simulink model "IMU2"  (R2018b)
settings: Solver=FixedStepAuto  StartTime=0.0  StopTime=inf  RelTol=1e-3  EnableMultiTasking=on
InitFcn:
  | Ts=0.1;
  | Delay=5;
  | Sample_div=uint8(9);
  | Filter_BW=uint8(2);  %cutoff 92 Hz
  | Gy_Conf=uint8(0); %-250dps to 250 dps
  | Acc_Conf1=uint8(0);
  | Acc_Conf2=uint8(2);
  | FIFO_en=uint8(0); % Disabled
  | INT_en=uint8(0); % Disabled
  | Acc_Scale=2*9.81/32767;
  | 
  | %Registers
  | IMU_Add=104;
  | Who_Am_I=117;
  | PWR_1=107;
  | PWR_2=108;
  | SAMPL_DIV=25;
  | CONFIG_REG=26;
  | GYRO_CONFIG=27;
  | ACC_CONFIG_1=28;
  | ACC_CONFIG_2=29;
  | FIFO_EN=35;
  | INT_EN=56;
  | GY_X_OFFSET_H=19;
  | GY_X_OFFSET_L=20;
  | GY_Y_OFFSET_H=21;
  | GY_Y_OFFSET_L=22;
  | GY_Z_OFFSET_H=23;
  | GY_Z_OFFSET_L=24;
  | ACC_X_OFFSET_H=119;
  | ACC_X_OFFSET_L=120;
  | ACC_Y_OFFSET_H=122;
  | ACC_Y_OFFSET_L=123;
  | ACC_Z_OFFSET_H=125;
  | ACC_Z_OFFSET_L=126;
  | ACCEL_XOUT_H=59;
  | ACCEL_XOUT_L=60;
  | ACCEL_YOUT_H=61;
  | ACCEL_YOUT_L=62;
  | ACCEL_ZOUT_H=63;
  | ACCEL_ZOUT_L=64
libraries: arduinolib x14
settings Model: SimulationMode=external  ExtModeTrigDuration=2  Creator=amind  LastModifiedBy=PC WORLD
settings OptimizationCC: EnhancedBackFolding=on  PassReuseOutputArgsAs=Individual arguments  MaxStackSize=64  OptimizeBlockOrder=speed  DifferentSizesBufferReuse=on  OptimizationCustomize=off
settings DebuggingCC: ParameterPrecisionLossMsg=none  ParameterTunabilityLossMsg=error
settings HardwareCC: ProdBitPerInt=16  ProdBitPerPointer=16  ProdBitPerSizeT=16  ProdBitPerPtrDiffT=16  ProdLargestAtomicFloat=None  ProdWordSize=8  ProdHWDeviceType=Atmel->AVR
settings SFSimCC: MATLABDynamicMemAlloc=off
settings RTWCC: SystemTargetFile=ert.tlc  HardwareBoard=Arduino Mega 2560  TemplateMakefile=ert_default_tmf  GenerateReport=on  Toolchain=Arduino AVR  BuildConfiguration=Faster Runs  IncludeHyperlinkInReport=on  LaunchReport=on  GenerateTraceInfo=on  GenerateTraceReport=on  GenerateTraceReportSl=on  GenerateTraceReportSf=on  GenerateTraceReportEml=on
settings CodeAppCC: ForceParamTrailComments=on  IgnoreCustomStorageClasses=off  OperatorAnnotations=on  SimulinkDataObjDesc=on  SFDataObjDesc=on  InsertBlockDesc=on
settings ERTTargetCC: SupportContinuousTime=on  SupportVariableSizeSignals=on

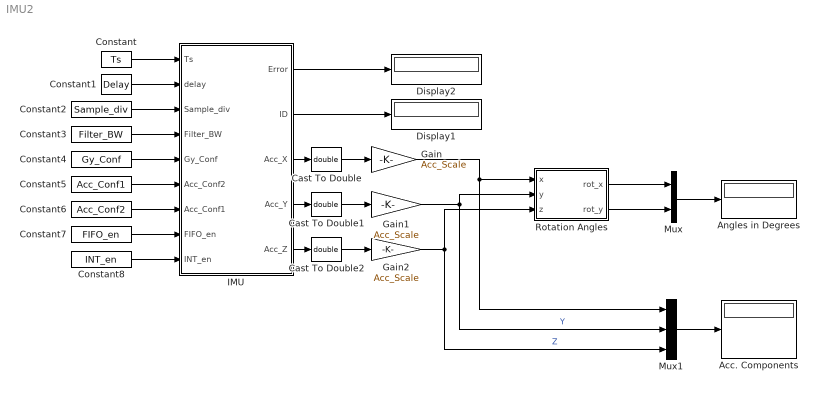
== system IMU2 ==
  Acc. Components : Display
  Angles in Degrees : Display
  Cast To Double : DataTypeConversion  OutDataTypeStr=double
  Cast To Double1 : DataTypeConversion  OutDataTypeStr=double
  Cast To Double2 : DataTypeConversion  OutDataTypeStr=double
  Constant : Constant  Value=Ts
  Constant1 : Constant  Value=Delay
  Constant2 : Constant  Value=Sample_div
  Constant3 : Constant  Value=Filter_BW
  Constant4 : Constant  Value=Gy_Conf
  Constant5 : Constant  Value=Acc_Conf1
  Constant6 : Constant  Value=Acc_Conf2
  Constant7 : Constant  Value=FIFO_en
  Constant8 : Constant  Value=INT_en
  Display1 : Display
  Display2 : Display
  Gain : Gain  Gain=Acc_Scale
  Gain1 : Gain  Gain=Acc_Scale
  Gain2 : Gain  Gain=Acc_Scale
  IMU : Stateflow chart  TreatAsAtomicUnit=on
  Mux : Mux  Inputs=2
  Mux1 : Mux  Inputs=3
  Rotation Angles : MATLAB Function  TreatAsAtomicUnit=on
  wires:
  IMU/1(Error) -> Display2/1
  IMU/2(ID) -> Display1/1
  Constant/1 -> IMU/1(Ts)
  Constant1/1 -> IMU/2(delay)
  Constant2/1 -> IMU/3(Sample_div)
  Constant3/1 -> IMU/4(Filter_BW)
  Constant4/1 -> IMU/5(Gy_Conf)
  Constant5/1 -> IMU/6(Acc_Conf2)
  Constant6/1 -> IMU/7(Acc_Conf1)
  Constant7/1 -> IMU/8(FIFO_en)
  Constant8/1 -> IMU/9(INT_en)
  IMU/3(Acc_X) -> Cast To Double/1
  IMU/4(Acc_Y) -> Cast To Double1/1
  IMU/5(Acc_Z) -> Cast To Double2/1
  Mux/1 -> Angles in Degrees/1
  Cast To Double/1 -> Gain/1
  Cast To Double1/1 -> Gain1/1
  Cast To Double2/1 -> Gain2/1
  Gain/1 -> Rotation Angles/1(x), Mux1/1
  Mux1/1 -> Acc. Components/1
  Gain2/1 -> Rotation Angles/3(z), Mux1/3  "Z"
  Gain1/1 -> Mux1/2, Rotation Angles/2(y)  "Y"
  Rotation Angles/1(rot_x) -> Mux/1
  Rotation Angles/2(rot_y) -> Mux/2

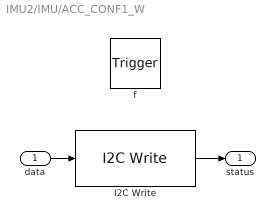
== system IMU2/IMU/ACC_CONF1_W ==
  data : Inport  OutDataTypeStr=uint8  PortDimensions=1
  f : TriggerPort  TriggerType=function-call  VariantControl=(inherit)
      settings: CopyFcn=Stateflow.SLINSF.SimulinkMan.removeBlockPreDeleteFcn  PreDeleteFcn=Stateflow.SLINSF.SimulinkMan.unsafePredeleteFcn
  I2C Write : arduinolib/I2C Write  I2CModule=0  Mode=Master  SlaveAddress=IMU_Add  SlaveByteOrder=BigEndian  Direction=Transmitter  RegisterAddressMode=on  RegisterAddress=ACC_CONFIG_1  SlaveDataType=uint8  DataLength=1  NoAck=off  RepeatedStart=off  OutputStatus=on  blockPlatform=ARDUINO
      settings: SourceProductName=Simulink Support Package for Arduino Hardware  SourceProductBaseCode=ARDUINO
  status : Outport  VectorParamsAs1DForOutWhenUnconnected=off
  wires:
  I2C Write/1 -> status/1
  data/1 -> I2C Write/1

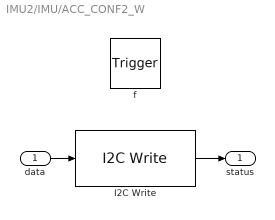
== system IMU2/IMU/ACC_CONF2_W ==
  data : Inport  OutDataTypeStr=uint8  PortDimensions=1
  f : TriggerPort  TriggerType=function-call  VariantControl=(inherit)
      settings: CopyFcn=Stateflow.SLINSF.SimulinkMan.removeBlockPreDeleteFcn  PreDeleteFcn=Stateflow.SLINSF.SimulinkMan.unsafePredeleteFcn
  I2C Write : arduinolib/I2C Write  I2CModule=0  Mode=Master  SlaveAddress=IMU_Add  SlaveByteOrder=BigEndian  Direction=Transmitter  RegisterAddressMode=on  RegisterAddress=ACC_CONFIG_2  SlaveDataType=uint8  DataLength=1  NoAck=off  RepeatedStart=off  OutputStatus=on  blockPlatform=ARDUINO
      settings: SourceProductName=Simulink Support Package for Arduino Hardware  SourceProductBaseCode=ARDUINO
  status : Outport  VectorParamsAs1DForOutWhenUnconnected=off
  wires:
  I2C Write/1 -> status/1
  data/1 -> I2C Write/1

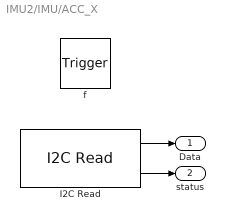
== system IMU2/IMU/ACC_X ==
  f : TriggerPort  TriggerType=function-call  VariantControl=(inherit)
      settings: CopyFcn=Stateflow.SLINSF.SimulinkMan.removeBlockPreDeleteFcn  PreDeleteFcn=Stateflow.SLINSF.SimulinkMan.unsafePredeleteFcn
  I2C Read : arduinolib/I2C Read  I2CModule=0  Mode=Master  SlaveAddress=IMU_Add  SlaveByteOrder=BigEndian  Direction=Receiver  RegisterAddressMode=on  RegisterAddress=ACCEL_XOUT_H  SlaveDataType=int16  DataLength=1  NoAck=off  RepeatedStart=off  OutputStatus=on  blockPlatform=ARDUINO  SampleTime=-1
      settings: SourceProductName=Simulink Support Package for Arduino Hardware  SourceProductBaseCode=ARDUINO
  Data : Outport  VectorParamsAs1DForOutWhenUnconnected=off
  status : Outport  Port=2  VectorParamsAs1DForOutWhenUnconnected=off
  wires:
  I2C Read/1 -> Data/1
  I2C Read/2 -> status/1

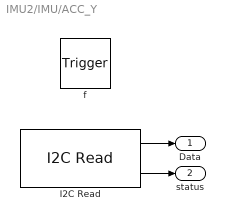
== system IMU2/IMU/ACC_Y ==
  f : TriggerPort  TriggerType=function-call  VariantControl=(inherit)
      settings: CopyFcn=Stateflow.SLINSF.SimulinkMan.removeBlockPreDeleteFcn  PreDeleteFcn=Stateflow.SLINSF.SimulinkMan.unsafePredeleteFcn
  I2C Read : arduinolib/I2C Read  I2CModule=0  Mode=Master  SlaveAddress=IMU_Add  SlaveByteOrder=BigEndian  Direction=Receiver  RegisterAddressMode=on  RegisterAddress=ACCEL_YOUT_H  SlaveDataType=int16  DataLength=1  NoAck=off  RepeatedStart=off  OutputStatus=on  blockPlatform=ARDUINO  SampleTime=-1
      settings: SourceProductName=Simulink Support Package for Arduino Hardware  SourceProductBaseCode=ARDUINO
  Data : Outport  VectorParamsAs1DForOutWhenUnconnected=off
  status : Outport  Port=2  VectorParamsAs1DForOutWhenUnconnected=off
  wires:
  I2C Read/1 -> Data/1
  I2C Read/2 -> status/1

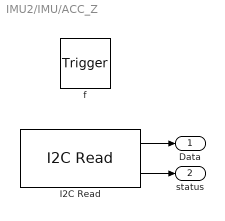
== system IMU2/IMU/ACC_Z ==
  f : TriggerPort  TriggerType=function-call  VariantControl=(inherit)
      settings: CopyFcn=Stateflow.SLINSF.SimulinkMan.removeBlockPreDeleteFcn  PreDeleteFcn=Stateflow.SLINSF.SimulinkMan.unsafePredeleteFcn
  I2C Read : arduinolib/I2C Read  I2CModule=0  Mode=Master  SlaveAddress=IMU_Add  SlaveByteOrder=BigEndian  Direction=Receiver  RegisterAddressMode=on  RegisterAddress=ACCEL_ZOUT_H  SlaveDataType=int16  DataLength=1  NoAck=off  RepeatedStart=off  OutputStatus=on  blockPlatform=ARDUINO  SampleTime=-1
      settings: SourceProductName=Simulink Support Package for Arduino Hardware  SourceProductBaseCode=ARDUINO
  Data : Outport  VectorParamsAs1DForOutWhenUnconnected=off
  status : Outport  Port=2  VectorParamsAs1DForOutWhenUnconnected=off
  wires:
  I2C Read/1 -> Data/1
  I2C Read/2 -> status/1

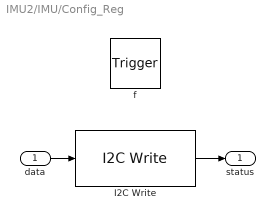
== system IMU2/IMU/Config_Reg ==
  data : Inport  OutDataTypeStr=uint8  PortDimensions=1
  f : TriggerPort  TriggerType=function-call  VariantControl=(inherit)
      settings: CopyFcn=Stateflow.SLINSF.SimulinkMan.removeBlockPreDeleteFcn  PreDeleteFcn=Stateflow.SLINSF.SimulinkMan.unsafePredeleteFcn
  I2C Write : arduinolib/I2C Write  I2CModule=0  Mode=Master  SlaveAddress=IMU_Add  SlaveByteOrder=BigEndian  Direction=Transmitter  RegisterAddressMode=on  RegisterAddress=CONFIG_REG  SlaveDataType=uint8  DataLength=1  NoAck=off  RepeatedStart=off  OutputStatus=on  blockPlatform=ARDUINO
      settings: SourceProductName=Simulink Support Package for Arduino Hardware  SourceProductBaseCode=ARDUINO
  status : Outport  VectorParamsAs1DForOutWhenUnconnected=off
  wires:
  I2C Write/1 -> status/1
  data/1 -> I2C Write/1

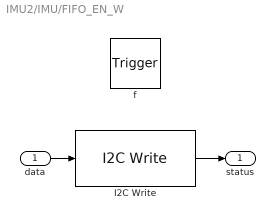
== system IMU2/IMU/FIFO_EN_W ==
  data : Inport  OutDataTypeStr=uint8  PortDimensions=1
  f : TriggerPort  TriggerType=function-call  VariantControl=(inherit)
      settings: CopyFcn=Stateflow.SLINSF.SimulinkMan.removeBlockPreDeleteFcn  PreDeleteFcn=Stateflow.SLINSF.SimulinkMan.unsafePredeleteFcn
  I2C Write : arduinolib/I2C Write  I2CModule=0  Mode=Master  SlaveAddress=IMU_Add  SlaveByteOrder=BigEndian  Direction=Transmitter  RegisterAddressMode=on  RegisterAddress=FIFO_EN  SlaveDataType=uint8  DataLength=1  NoAck=off  RepeatedStart=off  OutputStatus=on  blockPlatform=ARDUINO
      settings: SourceProductName=Simulink Support Package for Arduino Hardware  SourceProductBaseCode=ARDUINO
  status : Outport  VectorParamsAs1DForOutWhenUnconnected=off
  wires:
  I2C Write/1 -> status/1
  data/1 -> I2C Write/1

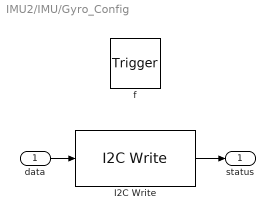
== system IMU2/IMU/Gyro_Config ==
  data : Inport  OutDataTypeStr=uint8  PortDimensions=1
  f : TriggerPort  TriggerType=function-call  VariantControl=(inherit)
      settings: CopyFcn=Stateflow.SLINSF.SimulinkMan.removeBlockPreDeleteFcn  PreDeleteFcn=Stateflow.SLINSF.SimulinkMan.unsafePredeleteFcn
  I2C Write : arduinolib/I2C Write  I2CModule=0  Mode=Master  SlaveAddress=IMU_Add  SlaveByteOrder=BigEndian  Direction=Transmitter  RegisterAddressMode=on  RegisterAddress=GYRO_CONFIG  SlaveDataType=uint8  DataLength=1  NoAck=off  RepeatedStart=off  OutputStatus=on  blockPlatform=ARDUINO
      settings: SourceProductName=Simulink Support Package for Arduino Hardware  SourceProductBaseCode=ARDUINO
  status : Outport  VectorParamsAs1DForOutWhenUnconnected=off
  wires:
  I2C Write/1 -> status/1
  data/1 -> I2C Write/1

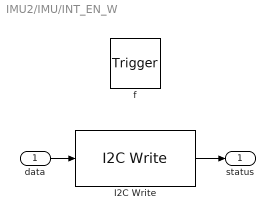
== system IMU2/IMU/INT_EN_W ==
  data : Inport  OutDataTypeStr=uint8  PortDimensions=1
  f : TriggerPort  TriggerType=function-call  VariantControl=(inherit)
      settings: CopyFcn=Stateflow.SLINSF.SimulinkMan.removeBlockPreDeleteFcn  PreDeleteFcn=Stateflow.SLINSF.SimulinkMan.unsafePredeleteFcn
  I2C Write : arduinolib/I2C Write  I2CModule=0  Mode=Master  SlaveAddress=IMU_Add  SlaveByteOrder=BigEndian  Direction=Transmitter  RegisterAddressMode=on  RegisterAddress=INT_EN  SlaveDataType=uint8  DataLength=1  NoAck=off  RepeatedStart=off  OutputStatus=on  blockPlatform=ARDUINO
      settings: SourceProductName=Simulink Support Package for Arduino Hardware  SourceProductBaseCode=ARDUINO
  status : Outport  VectorParamsAs1DForOutWhenUnconnected=off
  wires:
  I2C Write/1 -> status/1
  data/1 -> I2C Write/1

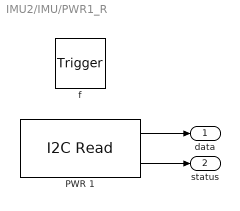
== system IMU2/IMU/PWR1_R ==
  f : TriggerPort  TriggerType=function-call  VariantControl=(inherit)
      settings: CopyFcn=Stateflow.SLINSF.SimulinkMan.removeBlockPreDeleteFcn  PreDeleteFcn=Stateflow.SLINSF.SimulinkMan.unsafePredeleteFcn
  PWR 1 : arduinolib/I2C Read  I2CModule=0  Mode=Master  SlaveAddress=IMU_Add  SlaveByteOrder=BigEndian  Direction=Receiver  RegisterAddressMode=on  RegisterAddress=PWR_1  SlaveDataType=uint8  DataLength=1  NoAck=off  RepeatedStart=off  OutputStatus=on  blockPlatform=ARDUINO  SampleTime=-1
      settings: SourceProductName=Simulink Support Package for Arduino Hardware  SourceProductBaseCode=ARDUINO
  data : Outport  VectorParamsAs1DForOutWhenUnconnected=off
  status : Outport  Port=2  VectorParamsAs1DForOutWhenUnconnected=off
  wires:
  PWR 1/1 -> data/1
  PWR 1/2 -> status/1

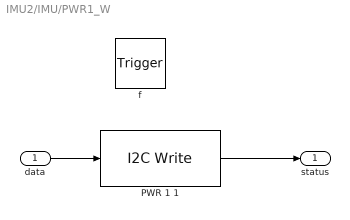
== system IMU2/IMU/PWR1_W ==
  data : Inport  OutDataTypeStr=uint8  PortDimensions=1
  f : TriggerPort  TriggerType=function-call  VariantControl=(inherit)
      settings: CopyFcn=Stateflow.SLINSF.SimulinkMan.removeBlockPreDeleteFcn  PreDeleteFcn=Stateflow.SLINSF.SimulinkMan.unsafePredeleteFcn
  PWR 1 1 : arduinolib/I2C Write  I2CModule=0  Mode=Master  SlaveAddress=IMU_Add  SlaveByteOrder=BigEndian  Direction=Transmitter  RegisterAddressMode=on  RegisterAddress=PWR_1  SlaveDataType=uint8  DataLength=1  NoAck=off  RepeatedStart=off  OutputStatus=on  blockPlatform=ARDUINO
      settings: SourceProductName=Simulink Support Package for Arduino Hardware  SourceProductBaseCode=ARDUINO
  status : Outport  VectorParamsAs1DForOutWhenUnconnected=off
  wires:
  data/1 -> PWR 1 1/1
  PWR 1 1/1 -> status/1

== system IMU2/IMU/PWR2_W ==
  data : Inport  OutDataTypeStr=uint8  PortDimensions=1
  f : TriggerPort  TriggerType=function-call  VariantControl=(inherit)
      settings: CopyFcn=Stateflow.SLINSF.SimulinkMan.removeBlockPreDeleteFcn  PreDeleteFcn=Stateflow.SLINSF.SimulinkMan.unsafePredeleteFcn
  I2C Write : arduinolib/I2C Write  I2CModule=0  Mode=Master  SlaveAddress=IMU_Add  SlaveByteOrder=BigEndian  Direction=Transmitter  RegisterAddressMode=on  RegisterAddress=PWR_2  SlaveDataType=uint8  DataLength=1  NoAck=off  RepeatedStart=off  OutputStatus=on  blockPlatform=ARDUINO
      settings: SourceProductName=Simulink Support Package for Arduino Hardware  SourceProductBaseCode=ARDUINO
  status : Outport  VectorParamsAs1DForOutWhenUnconnected=off
  wires:
  data/1 -> I2C Write/1
  I2C Write/1 -> status/1

== system IMU2/IMU/SAMPL_Div ==
  data : Inport  OutDataTypeStr=uint8  PortDimensions=1
  f : TriggerPort  TriggerType=function-call  VariantControl=(inherit)
      settings: CopyFcn=Stateflow.SLINSF.SimulinkMan.removeBlockPreDeleteFcn  PreDeleteFcn=Stateflow.SLINSF.SimulinkMan.unsafePredeleteFcn
  I2C Write : arduinolib/I2C Write  I2CModule=0  Mode=Master  SlaveAddress=IMU_Add  SlaveByteOrder=BigEndian  Direction=Transmitter  RegisterAddressMode=on  RegisterAddress=SAMPL_DIV  SlaveDataType=uint8  DataLength=1  NoAck=off  RepeatedStart=off  OutputStatus=on  blockPlatform=ARDUINO
      settings: SourceProductName=Simulink Support Package for Arduino Hardware  SourceProductBaseCode=ARDUINO
  status : Outport  VectorParamsAs1DForOutWhenUnconnected=off
  wires:
  I2C Write/1 -> status/1
  data/1 -> I2C Write/1

== system IMU2/IMU/Stop ==
  f : TriggerPort  TriggerType=function-call  VariantControl=(inherit)
      settings: CopyFcn=Stateflow.SLINSF.SimulinkMan.removeBlockPreDeleteFcn  PreDeleteFcn=Stateflow.SLINSF.SimulinkMan.unsafePredeleteFcn
  Constant : Constant
  Stop Simulation : Stop
  wires:
  Constant/1 -> Stop Simulation/1

== system IMU2/IMU/Who_Am_I ==
  f : TriggerPort  TriggerType=function-call  VariantControl=(inherit)
      settings: CopyFcn=Stateflow.SLINSF.SimulinkMan.removeBlockPreDeleteFcn  PreDeleteFcn=Stateflow.SLINSF.SimulinkMan.unsafePredeleteFcn
  I2C Read : arduinolib/I2C Read  I2CModule=0  Mode=Master  SlaveAddress=IMU_Add  SlaveByteOrder=BigEndian  Direction=Receiver  RegisterAddressMode=on  RegisterAddress=Who_Am_I  SlaveDataType=uint8  DataLength=1  NoAck=off  RepeatedStart=off  OutputStatus=on  blockPlatform=ARDUINO  SampleTime=-1
      settings: SourceProductName=Simulink Support Package for Arduino Hardware  SourceProductBaseCode=ARDUINO
  data : Outport  VectorParamsAs1DForOutWhenUnconnected=off
  status : Outport  Port=2  VectorParamsAs1DForOutWhenUnconnected=off
  wires:
  I2C Read/2 -> status/1
  I2C Read/1 -> data/1

== matlab function IMU2/Rotation Angles ==
  data: x input; rot_x output; y input; z input; rot_y output
function [rot_x,rot_y] = fcn(x,y,z)
  th=0.1;
  nor=sqrt(x^2+y^2+z^2);
  if(nor==0)
      nor=1;
  end
  x=x/nor;
  y=y/nor;
  z=z/nor;
  if(abs(x)<=th)
      x=0;
  end
  if(abs(y)<=th)
      y=0;
  end
  if(abs(z)<=th)
      z=0;
  end
  rot_x=atan2(y,z)*180/pi;
  rot_y=atan2(-x,sqrt(y^2+z^2))*180/pi;
 end

== stateflow chart IMU2/IMU ==
  state Stop [function]
  state [data,status] = Who_Am_I [function]
  state [data,status] = PWR1_R [function]
  state status=PWR1_W(data) [function]
  state status=PWR2_W(data) [function]
  state status = SAMPL_Div(data) [function]
  state status = Config_Reg(data) [function]
  state Measurments
    en:
    status=uint8(1);
    status1=uint8(1);
    status2=uint8(1);
    state ACC_X
      du:
      [Acc_X,status] = ACC_X;
    state ACC_Y
      du:
      [ Acc_Y,status1] = ACC_Y;
    state ACC_Z
      du:
      [Acc_Z,status2] = ACC_Z;
    (default) -> ACC_X
    ACC_X -> ACC_Y : [status==0]
    ACC_Y -> ACC_Z : [status1==0]
  state PWR_Adj
    en:
    status=uint8(1);
    status1=uint8(1);
    status2=uint8(1);
    state PWR1_R
      du:
      [data,status]=PWR1_R();
    state PWR1_W
      du:
      status1=PWR1_W(uint8(and(5,data)));
    state PWR2_W1
      du:
      status2= PWR2_W(uint8(0));
    (default) -> PWR1_R
    PWR1_R -> PWR1_W : [status==0]
    PWR1_W -> PWR2_W1 : [status1==0]
  state status = Gyro_Config(data) [function]
  state Acc_Conf
    en:
    status=uint8(1);
    status1=uint8(1);
    state ACC_Conf1
      du:
      status = ACC_CONF1_W(Acc_Conf1);
    state ACC_Conf2
      du:
      status1 = ACC_CONF2_W(Acc_Conf2);
    (default) -> ACC_Conf1
    ACC_Conf1 -> ACC_Conf2 : [status==0]
  state status = ACC_CONF1_W(data) [function]
  state status = ACC_CONF2_W(data) [function]
  state INT
    en:
    status=uint8(1);
    du:
    status=INT_EN_W(INT_en);
  state FIFO
    en:
    status=uint8(1);
    du:
    status=FIFO_EN_W(FIFO_en);
  state SAMPL_Rate_Div
    en:
    status=uint8(1);
    du:
    status=SAMPL_Div(Sample_div);
  state Config
    en:
    status=uint8(1);
    du:
    status = Config_Reg(Filter_BW);
  state Gyro_Conf
    en:
    status=uint8(1);
    du:
    status=Gyro_Config(Gy_Conf);
  state Identification
    en:
    status=uint8(1);
    du:
    [data,status]=Who_Am_I();
    ID=data;
  state status = FIFO_EN_W(data) [function]
  state status = INT_EN_W(data) [function]
  state [Data,status] = ACC_X [function]
  state [Data,status] = ACC_Y [function]
  state [Data,status] = ACC_Z [function]
  state Stopping
    en:
    Error=status;
    Stop();
  PWR_Adj -> SAMPL_Rate_Div [order 2] : [status==0 && status1==0 && status2==0]
  Acc_Conf -> FIFO [order 2] : [status==0 && status1==0]
  (default) -> Identification
  Measurments -> (junction 199) [order 1] : [status==0 && status1==0 && status2==0]
  INT -> Measurments [order 1] : [status==0]
  FIFO -> INT [order 2] : [status==0]
  SAMPL_Rate_Div -> Config [order 2] : [status==0]
  Config -> Gyro_Conf [order 2] : [status==0]
  Gyro_Conf -> Acc_Conf [order 2] : [status==0]
  (junction 199) -> Measurments : after(Ts,sec)
  Identification -> PWR_Adj [order 1] : [status==0 && data==113]
  SAMPL_Rate_Div -> Stopping [order 1] : after(delay,sec)
  FIFO -> Stopping [order 1] : after(delay,sec)
  INT -> Stopping [order 2] : after(delay,sec)
  Config -> Stopping [order 1] : after(delay,sec)
  Gyro_Conf -> Stopping [order 1] : after(delay,sec)
  Identification -> Stopping [order 2] : after(delay,sec)
  Acc_Conf -> Stopping [order 1] : after(delay,sec)
  PWR_Adj -> Stopping [order 1] : after(delay,sec)
  Measurments -> Stopping [order 2] : after(delay,sec)
  data: data function_output; status function_output; data function_output; status function_output; data function_input uint8 size=1; status function_output; data function_input uint8 size=1; status function_output; data function_input uint8 size=1; status function_output; data function_input uint8 size=1; status function_output; data function_input uint8 size=1; status function_output; data function_input uint8 size=1; status function_output; data function_input uint8 size=1; status function_output; data function_input uint8 size=1; status function_output; data function_input uint8 size=1; status function_output; Data function_output; status function_output; Data function_output; status function_output; Data function_output; status function_output; Error output; data local; status local; ID output; Acc_X output; Acc_Y output; Ts input; delay input; Sample_div input; Filter_BW input; Gy_Conf input; Acc_Conf2 input; Acc_Conf1 input; FIFO_en input; INT_en input; Acc_Z output; scale local; temp local; status2 local; status1 local
